simulink model "PTControl"  (Simulink 10.3)
settings: Solver=ode45  StartTime=0.0  StopTime=inf  RelTol=1e-3  EnableMultiTasking=on
(part 5 of 5)

== system PTControl/CarMaker/IPG Vehicle/PowerTrain/PTControl Example/PTControl_In/CreateBus PTC_Cfg Gearbox8 ==
  In : Inport
  BusCreator : BusCreator  Inputs=38
  Demux : Demux  Outputs=38
      settings: DisplayOption=none
  Out : Outport  VectorParamsAs1DForOutWhenUnconnected=off
  wires:
  Demux/38 -> BusCreator/38  "PTC_Cfg Gearbox8 iBGear16"
  Demux/37 -> BusCreator/37  "PTC_Cfg Gearbox8 iBGear15"
  Demux/36 -> BusCreator/36  "PTC_Cfg Gearbox8 iBGear14"
  Demux/35 -> BusCreator/35  "PTC_Cfg Gearbox8 iBGear13"
  Demux/34 -> BusCreator/34  "PTC_Cfg Gearbox8 iBGear12"
  Demux/33 -> BusCreator/33  "PTC_Cfg Gearbox8 iBGear11"
  Demux/32 -> BusCreator/32  "PTC_Cfg Gearbox8 iBGear10"
  Demux/31 -> BusCreator/31  "PTC_Cfg Gearbox8 iBGear9"
  Demux/30 -> BusCreator/30  "PTC_Cfg Gearbox8 iBGear8"
  Demux/29 -> BusCreator/29  "PTC_Cfg Gearbox8 iBGear7"
  Demux/28 -> BusCreator/28  "PTC_Cfg Gearbox8 iBGear6"
  Demux/27 -> BusCreator/27  "PTC_Cfg Gearbox8 iBGear5"
  Demux/26 -> BusCreator/26  "PTC_Cfg Gearbox8 iBGear4"
  Demux/25 -> BusCreator/25  "PTC_Cfg Gearbox8 iBGear3"
  Demux/24 -> BusCreator/24  "PTC_Cfg Gearbox8 iBGear2"
  Demux/23 -> BusCreator/23  "PTC_Cfg Gearbox8 iBGear1"
  Demux/22 -> BusCreator/22  "PTC_Cfg Gearbox8 iBGear0"
  Demux/21 -> BusCreator/21  "PTC_Cfg Gearbox8 nBGears"
  Demux/20 -> BusCreator/20  "PTC_Cfg Gearbox8 iFGear16"
  Demux/19 -> BusCreator/19  "PTC_Cfg Gearbox8 iFGear15"
  Demux/18 -> BusCreator/18  "PTC_Cfg Gearbox8 iFGear14"
  Demux/17 -> BusCreator/17  "PTC_Cfg Gearbox8 iFGear13"
  Demux/16 -> BusCreator/16  "PTC_Cfg Gearbox8 iFGear12"
  Demux/15 -> BusCreator/15  "PTC_Cfg Gearbox8 iFGear11"
  Demux/14 -> BusCreator/14  "PTC_Cfg Gearbox8 iFGear10"
  Demux/13 -> BusCreator/13  "PTC_Cfg Gearbox8 iFGear9"
  Demux/12 -> BusCreator/12  "PTC_Cfg Gearbox8 iFGear8"
  Demux/11 -> BusCreator/11  "PTC_Cfg Gearbox8 iFGear7"
  Demux/10 -> BusCreator/10  "PTC_Cfg Gearbox8 iFGear6"
  Demux/9 -> BusCreator/9  "PTC_Cfg Gearbox8 iFGear5"
  Demux/8 -> BusCreator/8  "PTC_Cfg Gearbox8 iFGear4"
  Demux/7 -> BusCreator/7  "PTC_Cfg Gearbox8 iFGear3"
  Demux/6 -> BusCreator/6  "PTC_Cfg Gearbox8 iFGear2"
  Demux/5 -> BusCreator/5  "PTC_Cfg Gearbox8 iFGear1"
  Demux/4 -> BusCreator/4  "PTC_Cfg Gearbox8 iFGear0"
  Demux/3 -> BusCreator/3  "PTC_Cfg Gearbox8 nFGears"
  Demux/2 -> BusCreator/2  "PTC_Cfg Gearbox8 ClKind"
  Demux/1 -> BusCreator/1  "PTC_Cfg Gearbox8 GBKind"
  BusCreator/1 -> Out/1
  In/1 -> Demux/1

== system PTControl/CarMaker/IPG Vehicle/PowerTrain/PTControl Example/PTControl_In/CreateBus PTC_Cfg Gearbox9 ==
  In : Inport
  BusCreator : BusCreator  Inputs=38
  Demux : Demux  Outputs=38
      settings: DisplayOption=none
  Out : Outport  VectorParamsAs1DForOutWhenUnconnected=off
  wires:
  Demux/38 -> BusCreator/38  "PTC_Cfg Gearbox9 iBGear16"
  Demux/37 -> BusCreator/37  "PTC_Cfg Gearbox9 iBGear15"
  Demux/36 -> BusCreator/36  "PTC_Cfg Gearbox9 iBGear14"
  Demux/35 -> BusCreator/35  "PTC_Cfg Gearbox9 iBGear13"
  Demux/34 -> BusCreator/34  "PTC_Cfg Gearbox9 iBGear12"
  Demux/33 -> BusCreator/33  "PTC_Cfg Gearbox9 iBGear11"
  Demux/32 -> BusCreator/32  "PTC_Cfg Gearbox9 iBGear10"
  Demux/31 -> BusCreator/31  "PTC_Cfg Gearbox9 iBGear9"
  Demux/30 -> BusCreator/30  "PTC_Cfg Gearbox9 iBGear8"
  Demux/29 -> BusCreator/29  "PTC_Cfg Gearbox9 iBGear7"
  Demux/28 -> BusCreator/28  "PTC_Cfg Gearbox9 iBGear6"
  Demux/27 -> BusCreator/27  "PTC_Cfg Gearbox9 iBGear5"
  Demux/26 -> BusCreator/26  "PTC_Cfg Gearbox9 iBGear4"
  Demux/25 -> BusCreator/25  "PTC_Cfg Gearbox9 iBGear3"
  Demux/24 -> BusCreator/24  "PTC_Cfg Gearbox9 iBGear2"
  Demux/23 -> BusCreator/23  "PTC_Cfg Gearbox9 iBGear1"
  Demux/22 -> BusCreator/22  "PTC_Cfg Gearbox9 iBGear0"
  Demux/21 -> BusCreator/21  "PTC_Cfg Gearbox9 nBGears"
  Demux/20 -> BusCreator/20  "PTC_Cfg Gearbox9 iFGear16"
  Demux/19 -> BusCreator/19  "PTC_Cfg Gearbox9 iFGear15"
  Demux/18 -> BusCreator/18  "PTC_Cfg Gearbox9 iFGear14"
  Demux/17 -> BusCreator/17  "PTC_Cfg Gearbox9 iFGear13"
  Demux/16 -> BusCreator/16  "PTC_Cfg Gearbox9 iFGear12"
  Demux/15 -> BusCreator/15  "PTC_Cfg Gearbox9 iFGear11"
  Demux/14 -> BusCreator/14  "PTC_Cfg Gearbox9 iFGear10"
  Demux/13 -> BusCreator/13  "PTC_Cfg Gearbox9 iFGear9"
  Demux/12 -> BusCreator/12  "PTC_Cfg Gearbox9 iFGear8"
  Demux/11 -> BusCreator/11  "PTC_Cfg Gearbox9 iFGear7"
  Demux/10 -> BusCreator/10  "PTC_Cfg Gearbox9 iFGear6"
  Demux/9 -> BusCreator/9  "PTC_Cfg Gearbox9 iFGear5"
  Demux/8 -> BusCreator/8  "PTC_Cfg Gearbox9 iFGear4"
  Demux/7 -> BusCreator/7  "PTC_Cfg Gearbox9 iFGear3"
  Demux/6 -> BusCreator/6  "PTC_Cfg Gearbox9 iFGear2"
  Demux/5 -> BusCreator/5  "PTC_Cfg Gearbox9 iFGear1"
  Demux/4 -> BusCreator/4  "PTC_Cfg Gearbox9 iFGear0"
  Demux/3 -> BusCreator/3  "PTC_Cfg Gearbox9 nFGears"
  Demux/2 -> BusCreator/2  "PTC_Cfg Gearbox9 ClKind"
  Demux/1 -> BusCreator/1  "PTC_Cfg Gearbox9 GBKind"
  BusCreator/1 -> Out/1
  In/1 -> Demux/1

== system PTControl/CarMaker/IPG Vehicle/PowerTrain/PTControl Example/PTControl_In/CreateBus PTC_Cfg ISG1 ==
  In : Inport
  BusCreator : BusCreator  Inputs=4
  Demux : Demux
      settings: DisplayOption=none
  Out : Outport  VectorParamsAs1DForOutWhenUnconnected=off
  wires:
  Demux/4 -> BusCreator/4  "PTC_Cfg ISG rotv_Gen_max"
  Demux/3 -> BusCreator/3  "PTC_Cfg ISG rotv_Mot_max"
  Demux/2 -> BusCreator/2  "PTC_Cfg ISG Ratio"
  Demux/1 -> BusCreator/1  "PTC_Cfg ISG Level"
  BusCreator/1 -> Out/1
  In/1 -> Demux/1

== system PTControl/CarMaker/IPG Vehicle/PowerTrain/PTControl Example/PTControl_In/CreateBus PTC_Cfg Misc1 ==
  In : Inport
  BusCreator : BusCreator  Inputs=14
  Demux : Demux  Outputs=14
      settings: DisplayOption=none
  Out : Outport  VectorParamsAs1DForOutWhenUnconnected=off
  wires:
  BusCreator/1 -> Out/1
  In/1 -> Demux/1
  Demux/4 -> BusCreator/4  "PTC_Cfg nClutch"
  Demux/11 -> BusCreator/11  "PTC_Cfg DriveSourcePos0"
  Demux/12 -> BusCreator/12  "PTC_Cfg DriveSourcePos1"
  Demux/14 -> BusCreator/14  "PTC_Cfg DriveSourcePos3"
  Demux/5 -> BusCreator/5  "PTC_Cfg nGearbox"
  Demux/2 -> BusCreator/2  "PTC_Cfg ClKind"
  Demux/10 -> BusCreator/10  "PTC_Cfg DL_iDiff_mean"
  Demux/9 -> BusCreator/9  "PTC_Cfg Aero_Frcx"
  Demux/1 -> BusCreator/1  "PTC_Cfg PTKind"
  Demux/8 -> BusCreator/8  "PTC_Cfg WheelRadius"
  Demux/13 -> BusCreator/13  "PTC_Cfg DriveSourcePos2"
  Demux/7 -> BusCreator/7  "PTC_Cfg Vehicle_nWheels"
  Demux/3 -> BusCreator/3  "PTC_Cfg nMotor"
  Demux/6 -> BusCreator/6  "PTC_Cfg nPlanetGear"

== system PTControl/CarMaker/IPG Vehicle/PowerTrain/PTControl Example/PTControl_In/CreateBus PTC_Cfg Motor1 ==
  In : Inport
  BusCreator : BusCreator  Inputs=48
  Demux : Demux  Outputs=48
      settings: DisplayOption=none
  Out : Outport  VectorParamsAs1DForOutWhenUnconnected=off
  wires:
  Demux/16 -> BusCreator/16  "PTC_Cfg Motor3 rotv_Gen_max"
  Demux/15 -> BusCreator/15  "PTC_Cfg Motor3 rotv_Mot_max"
  Demux/14 -> BusCreator/14  "PTC_Cfg Motor3 Ratio"
  Demux/13 -> BusCreator/13  "PTC_Cfg Motor3 Level"
  Demux/12 -> BusCreator/12  "PTC_Cfg Motor2 rotv_Gen_max"
  Demux/11 -> BusCreator/11  "PTC_Cfg Motor2 rotv_Mot_max"
  Demux/10 -> BusCreator/10  "PTC_Cfg Motor2 Ratio"
  Demux/9 -> BusCreator/9  "PTC_Cfg Motor2 Level"
  Demux/8 -> BusCreator/8  "PTC_Cfg Motor1 rotv_Gen_max"
  Demux/7 -> BusCreator/7  "PTC_Cfg Motor1 rotv_Mot_max"
  Demux/6 -> BusCreator/6  "PTC_Cfg Motor1 Ratio"
  Demux/5 -> BusCreator/5  "PTC_Cfg Motor1 Level"
  Demux/4 -> BusCreator/4  "PTC_Cfg Motor0 rotv_Gen_max"
  Demux/3 -> BusCreator/3  "PTC_Cfg Motor0 rotv_Mot_max"
  Demux/2 -> BusCreator/2  "PTC_Cfg Motor0 Ratio"
  Demux/1 -> BusCreator/1  "PTC_Cfg Motor0 Level"
  BusCreator/1 -> Out/1
  In/1 -> Demux/1
  Demux/17 -> BusCreator/17  "PTC_Cfg Motor4 Level"
  Demux/18 -> BusCreator/18  "PTC_Cfg Motor4 Ratio"
  Demux/19 -> BusCreator/19  "PTC_Cfg Motor4 rotv_Mot_max"
  Demux/20 -> BusCreator/20  "PTC_Cfg Motor4 rotv_Gen_max"
  Demux/21 -> BusCreator/21  "PTC_Cfg Motor5 Level"
  Demux/22 -> BusCreator/22  "PTC_Cfg Motor5 Ratio"
  Demux/23 -> BusCreator/23  "PTC_Cfg Motor5 rotv_Mot_max"
  Demux/24 -> BusCreator/24  "PTC_Cfg Motor5 rotv_Gen_max"
  Demux/25 -> BusCreator/25  "PTC_Cfg Motor6 Level"
  Demux/26 -> BusCreator/26  "PTC_Cfg Motor6 Ratio"
  Demux/27 -> BusCreator/27  "PTC_Cfg Motor6 rotv_Mot_max"
  Demux/28 -> BusCreator/28  "PTC_Cfg Motor6 rotv_Gen_max"
  Demux/29 -> BusCreator/29  "PTC_Cfg Motor7 Level"
  Demux/30 -> BusCreator/30  "PTC_Cfg Motor7 Ratio"
  Demux/31 -> BusCreator/31  "PTC_Cfg Motor7 rotv_Mot_max"
  Demux/32 -> BusCreator/32  "PTC_Cfg Motor7 rotv_Gen_max"
  Demux/33 -> BusCreator/33  "PTC_Cfg Motor8 Level"
  Demux/34 -> BusCreator/34  "PTC_Cfg Motor8 Ratio"
  Demux/35 -> BusCreator/35  "PTC_Cfg Motor8 rotv_Mot_max"
  Demux/36 -> BusCreator/36  "PTC_Cfg Motor8 rotv_Gen_max"
  Demux/37 -> BusCreator/37  "PTC_Cfg Motor9 Level"
  Demux/38 -> BusCreator/38  "PTC_Cfg Motor9 Ratio"
  Demux/39 -> BusCreator/39  "PTC_Cfg Motor9 rotv_Mot_max"
  Demux/40 -> BusCreator/40  "PTC_Cfg Motor9 rotv_Gen_max"
  Demux/41 -> BusCreator/41  "PTC_Cfg Motor10 Level"
  Demux/42 -> BusCreator/42  "PTC_Cfg Motor10 Ratio"
  Demux/43 -> BusCreator/43  "PTC_Cfg Motor10 rotv_Mot_max"
  Demux/44 -> BusCreator/44  "PTC_Cfg Motor10 rotv_Gen_max"
  Demux/45 -> BusCreator/45  "PTC_Cfg Motor11 Level"
  Demux/46 -> BusCreator/46  "PTC_Cfg Motor11 Ratio"
  Demux/47 -> BusCreator/47  "PTC_Cfg Motor11 rotv_Mot_max"
  Demux/48 -> BusCreator/48  "PTC_Cfg Motor11 rotv_Gen_max"

== system PTControl/CarMaker/IPG Vehicle/PowerTrain/PTControl Example/PTControl_In/CreateBus PTC_Cfg PlanetGear1 ==
  In : Inport
  BusCreator : BusCreator  Inputs=1
  Demux : Demux  Outputs=1
      settings: DisplayOption=none
  Out : Outport  VectorParamsAs1DForOutWhenUnconnected=off
  wires:
  Demux/1 -> BusCreator/1  "PTC_Cfg PlanetGear0 Ratio"
  BusCreator/1 -> Out/1
  In/1 -> Demux/1
